simulink model "Channelizer_demo_panel"  (R2023b)
settings: Solver=VariableStepAuto  StartTime=0.0  StopTime=inf  RelTol=1e-3
PostLoadFcn:
  | TT = numerictype(1,16,15);
  | FF = fimath('RoundingMethod','Nearest','OverflowAction','Saturate');
  | mdl = channelizer_init(TT, FF);
  | channelizer = channelizer_model(mdl, TT, FF );
  | Ts = 16*(7/4)/8.75e9;
  | ch_filt_coef = rcosdesign(0.22,4,28,'normal');
  | ch_filt_coef = 28 * ch_filt_coef / sum(ch_filt_coef(:));
  | channelizer_demo_init;
values from neighbouring files (symbols this model uses):
  ch0_en = 0    [channelizer_demo_init.m]    (also in init.m)
  ch0_qam = 0    [channelizer_demo_init.m]    (also in init.m)
  ch0_swp = 0    [channelizer_demo_init.m]    (also in init.m)
  ch10_en = 0    [channelizer_demo_init.m]    (also in init.m)
  ch10_qam = 0    [channelizer_demo_init.m]    (also in init.m)
  ch10_swp = 0    [channelizer_demo_init.m]    (also in init.m)
  ch11_en = 0    [channelizer_demo_init.m]    (also in init.m)
  ch11_qam = 0    [channelizer_demo_init.m]    (also in init.m)
  ch11_swp = 0    [channelizer_demo_init.m]    (also in init.m)
  ch12_en = 0    [channelizer_demo_init.m]    (also in init.m)
  ch12_qam = 0    [channelizer_demo_init.m]    (also in init.m)
  ch12_swp = 0    [channelizer_demo_init.m]    (also in init.m)
  ch13_en = 0    [channelizer_demo_init.m]    (also in init.m)
  ch13_qam = 0    [channelizer_demo_init.m]    (also in init.m)
  ch13_swp = 0    [channelizer_demo_init.m]    (also in init.m)
  ch14_en = 0    [channelizer_demo_init.m]    (also in init.m)
  ch14_qam = 0    [channelizer_demo_init.m]    (also in init.m)
  ch14_swp = 0    [channelizer_demo_init.m]    (also in init.m)
  ch15_en = 0    [channelizer_demo_init.m]    (also in init.m)
  ch15_qam = 0    [channelizer_demo_init.m]    (also in init.m)
  ch15_swp = 0    [channelizer_demo_init.m]    (also in init.m)
  ch1_en = 1    [channelizer_demo_init.m]    (also in init.m)
  ch1_qam = 0    [channelizer_demo_init.m]    (also in init.m)
  ch1_swp = 0    [channelizer_demo_init.m]    (also in init.m)
  ch2_en = 1    [channelizer_demo_init.m]    (also in init.m)
  ch2_qam = 0    [channelizer_demo_init.m]    (also in init.m)
  ch2_swp = 0    [channelizer_demo_init.m]    (also in init.m)
  ch3_en = 0    [channelizer_demo_init.m]    (also in init.m)
  ch3_qam = 0    [channelizer_demo_init.m]    (also in init.m)
  ch3_swp = 0    [channelizer_demo_init.m]    (also in init.m)
  ch4_en = 0    [channelizer_demo_init.m]    (also in init.m)
  ch4_qam = 0    [channelizer_demo_init.m]    (also in init.m)
  ch4_swp = 0    [channelizer_demo_init.m]    (also in init.m)
  ch5_en = 1    [channelizer_demo_init.m]    (also in init.m)
  ch5_qam = 1    [channelizer_demo_init.m]    (also in init.m)
  ch5_swp = 0    [channelizer_demo_init.m]    (also in init.m)
  ch6_en = 1    [channelizer_demo_init.m]    (also in init.m)
  ch6_qam = 1    [channelizer_demo_init.m]    (also in init.m)
  ch6_swp = 0    [channelizer_demo_init.m]    (also in init.m)
  ch7_en = 0    [channelizer_demo_init.m]    (also in init.m)
  ch7_qam = 0    [channelizer_demo_init.m]    (also in init.m)
  ch7_swp = 0    [channelizer_demo_init.m]    (also in init.m)
  ch8_en = 0    [channelizer_demo_init.m]    (also in init.m)
  ch8_qam = 0    [channelizer_demo_init.m]    (also in init.m)
  ch8_swp = 0    [channelizer_demo_init.m]    (also in init.m)
  ch9_en = 0    [channelizer_demo_init.m]    (also in init.m)
  ch9_qam = 0    [channelizer_demo_init.m]    (also in init.m)
  ch9_swp = 0    [channelizer_demo_init.m]    (also in init.m)
  spec1_ch = 1    [channelizer_demo_init.m]    (also in init.m)
  spec2_ch = 2    [channelizer_demo_init.m]    (also in init.m)
  spec3_ch = 5    [channelizer_demo_init.m]    (also in init.m)
  spec4_ch = 6    [channelizer_demo_init.m]    (also in init.m)
  swp_rate0 = 0    [channelizer_demo_init.m]    (also in init.m)
  swp_rate1 = 0    [channelizer_demo_init.m]    (also in init.m)
  swp_rate10 = 0    [channelizer_demo_init.m]    (also in init.m)
  swp_rate11 = 0    [channelizer_demo_init.m]    (also in init.m)
  swp_rate12 = 0    [channelizer_demo_init.m]    (also in init.m)
  swp_rate13 = 0    [channelizer_demo_init.m]    (also in init.m)
  swp_rate14 = 0    [channelizer_demo_init.m]    (also in init.m)
  swp_rate15 = 0    [channelizer_demo_init.m]    (also in init.m)
  swp_rate2 = 0    [channelizer_demo_init.m]    (also in init.m)
  swp_rate3 = 0    [channelizer_demo_init.m]    (also in init.m)
  swp_rate4 = 0    [channelizer_demo_init.m]    (also in init.m)
  swp_rate5 = 0    [channelizer_demo_init.m]    (also in init.m)
  swp_rate6 = 0    [channelizer_demo_init.m]    (also in init.m)
  swp_rate7 = 0    [channelizer_demo_init.m]    (also in init.m)
  swp_rate8 = 0    [channelizer_demo_init.m]    (also in init.m)
  swp_rate9 = 0    [channelizer_demo_init.m]    (also in init.m)
undefined symbols (not defined in the file or in its folder): S, vsva2197, xcvc1902
libraries: aieUtilities x39, aieBasic x34, dspswit3 x16, dspsigops x16, hlsBasic x3, vmcUtilities x1, commchan3 x1
(part 5 of 5)

== system Channelizer_demo_panel/Wideband_Signal/Subsystem9 ==
  swp_en : Inport
  chan_fc : Inport  Port=2
  qam_sym : Inport  Port=3
  qam_en : Inport  Port=4
  chan_en : EnablePort
  Add1 : Sum
  Constant : Constant  Value=complex(ones(28,1))  SampleTime=-1
  Constant1 : Constant  Value=complex(zeros(27,1))  SampleTime=-1
  Counter : dspswit3/Counter  Direction=Up  CountEvent=Non-zero sample  CounterSize=User defined  MaxCount=2^31-1  InitialCount=0  Output=Count  HitValue=32  ResetInput=off  SamplesPerFrame=1  Ts=16*(7/4)/8.75e9  CntDtype=int32  HitDtype=Logical
  Discrete FIR Filter : DiscreteFir  Coefficients=ch_filt_coef  InputProcessing=Columns as channels (frame based)
  Gain7 : Gain  Gain=swp_rate8  ParamDataTypeStr=double  OutDataTypeStr=int32  SaturateOnIntegerOverflow=on
  Gain8 : Gain  Gain=2^12  OutDataTypeStr=int32
  Mux : Mux  Inputs=2
  NCO : dspsigops/NCO  AccIncSrc=Input port  AccInc=100  PhaseOffsetSrc=Specify via dialog  PhaseOffset=0  AccumWL=16  HasDither=on  DitherWL=4  PNgeneratorLength=19  HasPhaseQuantizer=on  TableDepth=12  HasOutputPhaseError=off  Formula=Complex exponential  DataType=double  OutputWL=16  OutputFL=14  CompMethod=Table lookup (no interpolation)  SampleTime=1  SamplesPerFrame=28  OutputFrames=off
      settings: LibrarySourceBlock=dspsrcs4/NCO
  Product : Product
  Switch : Switch  Criteria=u2 > Threshold  SaturateOnIntegerOverflow=off  InputSameDT=off
  chan_out : Outport  OutputWhenDisabled=reset  InitialOutput=zeros(28,1)
  wires:
  NCO/1 -> Product/1
  swp_en/1 -> Counter/1
  Add1/1 -> NCO/1
  Product/1 -> chan_out/1
  Gain8/1 -> Add1/2
  Counter/1 -> Gain7/1
  Gain7/1 -> Add1/1
  chan_fc/1 -> Gain8/1
  Switch/1 -> Product/2
  Discrete FIR Filter/1 -> Switch/1
  qam_en/1 -> Switch/2
  Constant/1 -> Switch/3
  Mux/1 -> Discrete FIR Filter/1
  qam_sym/1 -> Mux/1
  Constant1/1 -> Mux/2
